simulink model "chap04_CA2"  (R2021a)
settings: Solver=FixedStepDiscrete  StartTime=0.0  StopTime=30  FixedStep=0.001  RelTol=1e-3
undefined symbols (not defined in the file): DiscIntNeverNeededParam
libraries: simulink x4
(part 2 of 3)

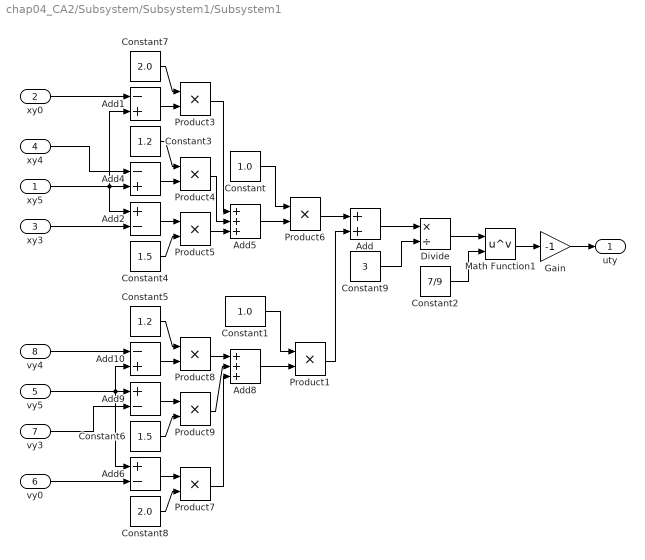
== system chap04_CA2/Subsystem/Subsystem1/Subsystem1 ==
  xy5 : Inport
  xy0 : Inport  Port=2
  xy3 : Inport  Port=3
  xy4 : Inport  Port=4
  vy5 : Inport  Port=5
  vy0 : Inport  Port=6
  vy3 : Inport  Port=7
  vy4 : Inport  Port=8
  Add : Sum
  Add1 : Sum  Inputs=-+
  Add10 : Sum  Inputs=-+
  Add2 : Sum  Inputs=+-
  Add4 : Sum  Inputs=-+
  Add5 : Sum  Inputs=+++
  Add6 : Sum  Inputs=+-
  Add8 : Sum  Inputs=+++
  Add9 : Sum  Inputs=+-
  Constant : Constant  Value=1.0
  Constant1 : Constant  Value=1.0
  Constant2 : Constant  Value=7/9
  Constant3 : Constant  Value=1.2
  Constant4 : Constant  Value=1.5
  Constant5 : Constant  Value=1.2
  Constant6 : Constant  Value=1.5
  Constant7 : Constant  Value=2.0
  Constant8 : Constant  Value=2.0
  Constant9 : Constant  Value=3
  Divide : Product  Inputs=*/
  Gain : Gain  Gain=-1
  Math Function1 : Math  Operator=pow  SignedPower=on  SaturateOnIntegerOverflow=on
  Product{1,3..9} (8 alike) : Product
  uty : Outport
  wires:
  vy0/1 -> Add6/2
  Constant8/1 -> Product7/2
  Add6/1 -> Product7/1
  Product7/1 -> Add8/3
  Product3/1 -> Add5/1
  xy0/1 -> Add1/1
  Add1/1 -> Product3/2
  Constant7/1 -> Product3/1
  Product9/1 -> Add8/2
  Product8/1 -> Add8/1
  Add9/1 -> Product9/1
  Constant6/1 -> Product9/2
  Add10/1 -> Product8/2
  Constant5/1 -> Product8/1
  Add8/1 -> Product1/2
  Product4/1 -> Add5/2
  Product5/1 -> Add5/3
  Constant3/1 -> Product4/1
  Add4/1 -> Product4/2
  xy5/1 -> Add2/1, Add4/2, Add1/2
  Constant4/1 -> Product5/2
  Product6/1 -> Add/1
  Constant/1 -> Product6/1
  Constant1/1 -> Product1/1
  Product1/1 -> Add/2
  Add2/1 -> Product5/1
  Add5/1 -> Product6/2
  xy4/1 -> Add4/1
  xy3/1 -> Add2/2
  vy3/1 -> Add9/2
  vy4/1 -> Add10/1
  vy5/1 -> Add9/1, Add6/1, Add10/2
  Math Function1/1 -> Gain/1
  Constant9/1 -> Divide/2
  Divide/1 -> Math Function1/1
  Add/1 -> Divide/1
  Constant2/1 -> Math Function1/2
  Gain/1 -> uty/1

== system chap04_CA2/Subsystem/Subsystem1/Subsystem10 ==
  utx : Inport
  uty : Inport  Port=2
  utz : Inport  Port=3
  Add : Sum
  Constant3 : Constant
  Constant4 : Constant  Value=0
  Data Store Memory : DataStoreMemory  DataStoreName=utkz5  ReadBeforeWriteMsg=warning  WriteAfterWriteMsg=warning  WriteAfterReadMsg=warning  ShowAdditionalParam=off
  Data Store Memory1 : DataStoreMemory  DataStoreName=utky5  ReadBeforeWriteMsg=warning  WriteAfterWriteMsg=warning  WriteAfterReadMsg=warning  ShowAdditionalParam=off
  Data Store Memory2 : DataStoreMemory  DataStoreName=utkx5  ReadBeforeWriteMsg=warning  WriteAfterWriteMsg=warning  WriteAfterReadMsg=warning  ShowAdditionalParam=off
  Data Store Memory3 : DataStoreMemory  DataStoreName=uc5  ReadBeforeWriteMsg=warning  WriteAfterWriteMsg=warning  WriteAfterReadMsg=warning  ShowAdditionalParam=off
  Data Store Read : DataStoreRead  DataStoreName=uc5  IndexOptions=Index vector (dialog)  Indices=1  OutputSizes=1
  Data Store Read1 : DataStoreRead  DataStoreName=utkz5  IndexOptions=Index vector (dialog)  Indices=1  OutputSizes=1
  Data Store Read2 : DataStoreRead  DataStoreName=utky5  IndexOptions=Index vector (dialog)  Indices=1  OutputSizes=1
  Data Store Read3 : DataStoreRead  DataStoreName=utkx5  IndexOptions=Index vector (dialog)  Indices=1  OutputSizes=1
  Data Store Write : DataStoreWrite  DataStoreName=uc5  IndexOptions=Index vector (dialog)  Indices=1  OutputSizes=1
  Data Store Write3 : DataStoreWrite  DataStoreName=utkx5  IndexOptions=Index vector (dialog)  Indices=1  OutputSizes=1
  Data Store Write4 : DataStoreWrite  DataStoreName=utky5  IndexOptions=Index vector (dialog)  Indices=1  OutputSizes=1
  Data Store Write5 : DataStoreWrite  DataStoreName=utkz5  IndexOptions=Index vector (dialog)  Indices=1  OutputSizes=1
  Demux : Demux  Outputs=3
  Display : Display
  MATLAB Function : MATLAB Function  TreatAsAtomicUnit=on
  Mux1 : Mux  Inputs=3
  Mux2 : Mux  Inputs=3
  Switch : Switch  Threshold=0.025
  Switch2 : Switch  Threshold=0.025
  ux : Outport
  uy : Outport  Port=2
  uz : Outport  Port=3
  wires:
  Mux2/1 -> [utk], MATLAB Function/2(utk)
  Mux1/1 -> [ut], MATLAB Function/1(u)
  Switch/1 -> Demux/1
  Data Store Read3/1 -> Mux2/1
  Data Store Read1/1 -> Mux2/3
  Data Store Read2/1 -> Mux2/2
  Demux/3 -> Data Store Write5/1, uz/1
  Demux/1 -> Data Store Write3/1, ux/1
  Add/1 -> Data Store Write/1, Display/1
  Data Store Read/1 -> Add/2
  Switch2/1 -> Add/1  "e1"
  Constant3/1 -> Switch2/1
  Constant4/1 -> Switch2/3
  MATLAB Function/1(nrom) -> Switch2/2, Switch/2
  utx/1 -> Mux1/1
  uty/1 -> Mux1/2
  utz/1 -> Mux1/3
  Demux/2 -> Data Store Write4/1, uy/1
  [ut] -> Switch/1
  [utk] -> Switch/3

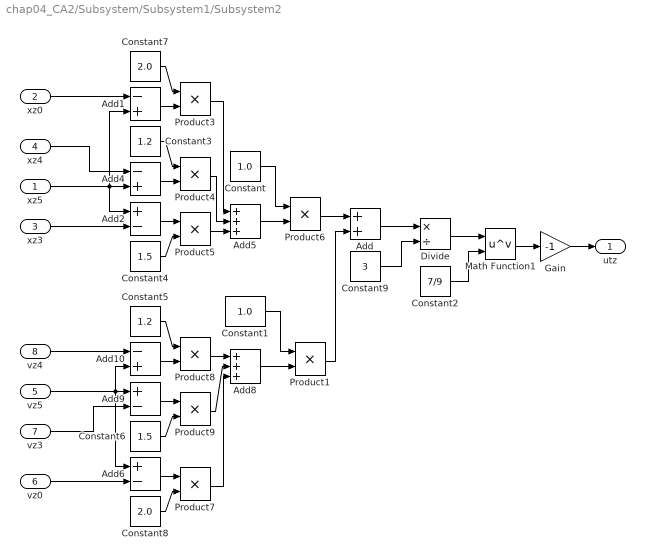
== system chap04_CA2/Subsystem/Subsystem1/Subsystem2 ==
  xz5 : Inport
  xz0 : Inport  Port=2
  xz3 : Inport  Port=3
  xz4 : Inport  Port=4
  vz5 : Inport  Port=5
  vz0 : Inport  Port=6
  vz3 : Inport  Port=7
  vz4 : Inport  Port=8
  Add : Sum
  Add1 : Sum  Inputs=-+
  Add10 : Sum  Inputs=-+
  Add2 : Sum  Inputs=+-
  Add4 : Sum  Inputs=-+
  Add5 : Sum  Inputs=+++
  Add6 : Sum  Inputs=+-
  Add8 : Sum  Inputs=+++
  Add9 : Sum  Inputs=+-
  Constant : Constant  Value=1.0
  Constant1 : Constant  Value=1.0
  Constant2 : Constant  Value=7/9
  Constant3 : Constant  Value=1.2
  Constant4 : Constant  Value=1.5
  Constant5 : Constant  Value=1.2
  Constant6 : Constant  Value=1.5
  Constant7 : Constant  Value=2.0
  Constant8 : Constant  Value=2.0
  Constant9 : Constant  Value=3
  Divide : Product  Inputs=*/
  Gain : Gain  Gain=-1
  Math Function1 : Math  Operator=pow  SignedPower=on  SaturateOnIntegerOverflow=on
  Product{1,3..9} (8 alike) : Product
  utz : Outport
  wires:
  vz5/1 -> Add10/2, Add6/1, Add9/1
  vz4/1 -> Add10/1
  vz3/1 -> Add9/2
  xz3/1 -> Add2/2
  xz4/1 -> Add4/1
  Add5/1 -> Product6/2
  Add2/1 -> Product5/1
  Product1/1 -> Add/2
  Constant1/1 -> Product1/1
  Constant/1 -> Product6/1
  Product6/1 -> Add/1
  Constant4/1 -> Product5/2
  xz5/1 -> Add1/2, Add4/2, Add2/1
  Add4/1 -> Product4/2
  Constant3/1 -> Product4/1
  Product5/1 -> Add5/3
  Product4/1 -> Add5/2
  Add8/1 -> Product1/2
  Constant5/1 -> Product8/1
  Add10/1 -> Product8/2
  Constant6/1 -> Product9/2
  Add9/1 -> Product9/1
  Product8/1 -> Add8/1
  Product9/1 -> Add8/2
  Constant7/1 -> Product3/1
  Add1/1 -> Product3/2
  xz0/1 -> Add1/1
  Product3/1 -> Add5/1
  Product7/1 -> Add8/3
  Add6/1 -> Product7/1
  Constant8/1 -> Product7/2
  vz0/1 -> Add6/2
  Math Function1/1 -> Gain/1
  Constant9/1 -> Divide/2
  Divide/1 -> Math Function1/1
  Add/1 -> Divide/1
  Constant2/1 -> Math Function1/2
  Gain/1 -> utz/1

== system chap04_CA2/Subsystem/Subsystem1/Subsystem4 ==
  vx5 : Inport
  vx0 : Inport  Port=2
  utx : Inport  Port=3
  gain : Inport  Port=4
  Add1 : Sum  Inputs=--+
  Constant : Constant  Value=0.08
  Constant2 : Constant  Value=15
  Product : Product
  Product1 : Product
  Product2 : Product
  Subsystem : Subsystem
  Subtract : Sum  Inputs=+--
  Tanh : Trigonometry  Operator=tanh
  ux : Outport
  wires:
  Add1/1 -> ux/1
  utx/1 -> [A], Subsystem/1(zt3)
  Subsystem/1(Out1) -> Subtract/3
  Product/1 -> Add1/2
  vx5/1 -> Subtract/1
  Product2/1 -> Tanh/1
  Tanh/1 -> Product/1
  gain/1 -> Product/2
  [A] -> Add1/3
  Constant2/1 -> Product2/2
  Product1/1 -> Add1/1
  Constant/1 -> Product1/1
  Subtract/1 -> Product1/2, Product2/1
  vx0/1 -> Subtract/2

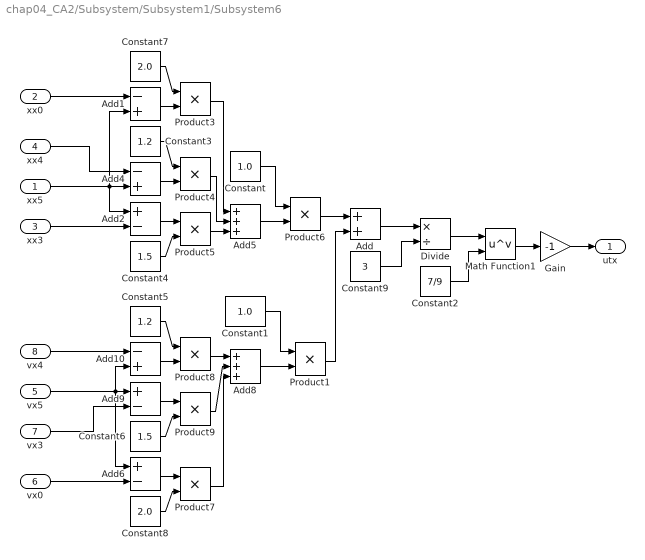
== system chap04_CA2/Subsystem/Subsystem1/Subsystem6 ==
  xx5 : Inport
  xx0 : Inport  Port=2
  xx3 : Inport  Port=3
  xx4 : Inport  Port=4
  vx5 : Inport  Port=5
  vx0 : Inport  Port=6
  vx3 : Inport  Port=7
  vx4 : Inport  Port=8
  Add : Sum
  Add1 : Sum  Inputs=-+
  Add10 : Sum  Inputs=-+
  Add2 : Sum  Inputs=+-
  Add4 : Sum  Inputs=-+
  Add5 : Sum  Inputs=+++
  Add6 : Sum  Inputs=+-
  Add8 : Sum  Inputs=+++
  Add9 : Sum  Inputs=+-
  Constant : Constant  Value=1.0
  Constant1 : Constant  Value=1.0
  Constant2 : Constant  Value=7/9
  Constant3 : Constant  Value=1.2
  Constant4 : Constant  Value=1.5
  Constant5 : Constant  Value=1.2
  Constant6 : Constant  Value=1.5
  Constant7 : Constant  Value=2.0
  Constant8 : Constant  Value=2.0
  Constant9 : Constant  Value=3
  Divide : Product  Inputs=*/
  Gain : Gain  Gain=-1
  Math Function1 : Math  Operator=pow  SignedPower=on  SaturateOnIntegerOverflow=on
  Product{1,3..9} (8 alike) : Product
  utx : Outport
  wires:
  vx5/1 -> Add10/2, Add6/1, Add9/1
  vx4/1 -> Add10/1
  vx3/1 -> Add9/2
  xx3/1 -> Add2/2
  xx4/1 -> Add4/1
  Add5/1 -> Product6/2
  Add2/1 -> Product5/1
  Product1/1 -> Add/2
  Constant1/1 -> Product1/1
  Constant/1 -> Product6/1
  Product6/1 -> Add/1
  Constant4/1 -> Product5/2
  xx5/1 -> Add1/2, Add4/2, Add2/1
  Add4/1 -> Product4/2
  Constant3/1 -> Product4/1
  Product5/1 -> Add5/3
  Product4/1 -> Add5/2
  Add8/1 -> Product1/2
  Constant5/1 -> Product8/1
  Add10/1 -> Product8/2
  Constant6/1 -> Product9/2
  Add9/1 -> Product9/1
  Product8/1 -> Add8/1
  Product9/1 -> Add8/2
  Constant7/1 -> Product3/1
  Add1/1 -> Product3/2
  xx0/1 -> Add1/1
  Product3/1 -> Add5/1
  Product7/1 -> Add8/3
  Add6/1 -> Product7/1
  Constant8/1 -> Product7/2
  vx0/1 -> Add6/2
  Math Function1/1 -> Gain/1
  Constant9/1 -> Divide/2
  Divide/1 -> Math Function1/1
  Add/1 -> Divide/1
  Constant2/1 -> Math Function1/2
  Gain/1 -> utx/1

== system chap04_CA2/Subsystem/Subsystem1/Subsystem7 ==
  vy5 : Inport
  vy0 : Inport  Port=2
  uty : Inport  Port=3
  gain : Inport  Port=4
  Add1 : Sum  Inputs=--+
  Constant : Constant  Value=0.08
  Constant2 : Constant  Value=15
  Product : Product
  Product1 : Product
  Product2 : Product
  Subsystem : Subsystem
  Subtract : Sum  Inputs=+--
  Tanh : Trigonometry  Operator=tanh
  ux : Outport
  wires:
  Subtract/1 -> Product2/1, Product1/2
  Constant/1 -> Product1/1
  Product1/1 -> Add1/1
  Constant2/1 -> Product2/2
  [A] -> Add1/3
  gain/1 -> Product/2
  Tanh/1 -> Product/1
  Product2/1 -> Tanh/1
  vy5/1 -> Subtract/1
  Product/1 -> Add1/2
  Subsystem/1(Out1) -> Subtract/3
  uty/1 -> Subsystem/1(zt3), [A]
  Add1/1 -> ux/1
  vy0/1 -> Subtract/2

== system chap04_CA2/Subsystem/Subsystem1/Subsystem8 ==
  vz5 : Inport
  vz0 : Inport  Port=2
  utz : Inport  Port=3
  gain : Inport  Port=4
  Add1 : Sum  Inputs=--+
  Constant : Constant  Value=0.08
  Constant2 : Constant  Value=15
  Product : Product
  Product1 : Product
  Product2 : Product
  Subsystem : Subsystem
  Subtract : Sum  Inputs=+--
  Tanh : Trigonometry  Operator=tanh
  ux : Outport
  wires:
  Add1/1 -> ux/1
  utz/1 -> [A], Subsystem/1(zt3)
  Subsystem/1(Out1) -> Subtract/3
  Product/1 -> Add1/2
  vz5/1 -> Subtract/1
  Product2/1 -> Tanh/1
  Tanh/1 -> Product/1
  gain/1 -> Product/2
  [A] -> Add1/3
  Constant2/1 -> Product2/2
  Product1/1 -> Add1/1
  Constant/1 -> Product1/1
  Subtract/1 -> Product1/2, Product2/1
  vz0/1 -> Subtract/2

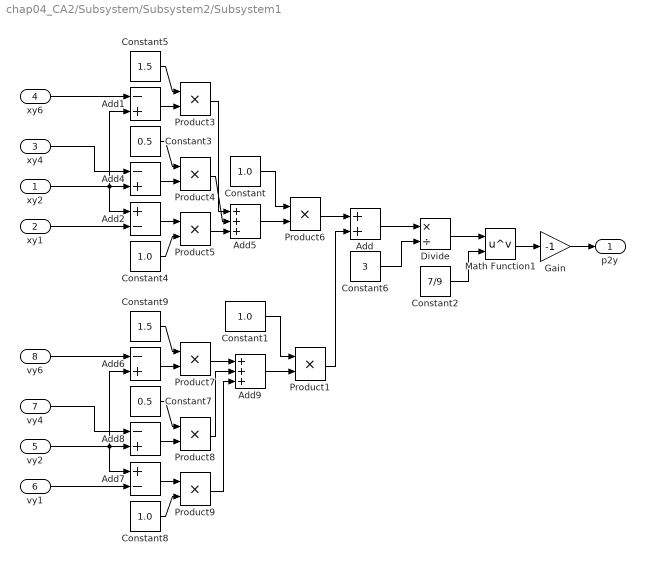
== system chap04_CA2/Subsystem/Subsystem2/Subsystem1 ==
  xy2 : Inport
  xy1 : Inport  Port=2
  xy4 : Inport  Port=3
  xy6 : Inport  Port=4
  vy2 : Inport  Port=5
  vy1 : Inport  Port=6
  vy4 : Inport  Port=7
  vy6 : Inport  Port=8
  Add : Sum
  Add{1,4,6,8} (4 alike) : Sum  Inputs=-+
  Add2 : Sum  Inputs=+-
  Add5 : Sum  Inputs=+++
  Add7 : Sum  Inputs=+-
  Add9 : Sum  Inputs=+++
  Constant{,1,4,8} (4 alike) : Constant  Value=1.0
  Constant2 : Constant  Value=7/9
  Constant3 : Constant  Value=0.5
  Constant5 : Constant  Value=1.5
  Constant6 : Constant  Value=3
  Constant7 : Constant  Value=0.5
  Constant9 : Constant  Value=1.5
  Divide : Product  Inputs=*/
  Gain : Gain  Gain=-1
  Math Function1 : Math  Operator=pow  SignedPower=on  SaturateOnIntegerOverflow=on
  Product{1,3..9} (8 alike) : Product
  p2y : Outport
  wires:
  Product8/1 -> Add9/2
  Product9/1 -> Add9/3
  Constant7/1 -> Product8/1
  Add8/1 -> Product8/2
  vy2/1 -> Add6/2, Add8/2, Add7/1
  Constant8/1 -> Product9/2
  Add7/1 -> Product9/1
  vy4/1 -> Add8/1
  vy1/1 -> Add7/2
  vy6/1 -> Add6/1
  Constant9/1 -> Product7/1
  Add6/1 -> Product7/2
  Product7/1 -> Add9/1
  Product3/1 -> Add5/1
  Add1/1 -> Product3/2
  Constant5/1 -> Product3/1
  xy6/1 -> Add1/1
  xy1/1 -> Add2/2
  xy4/1 -> Add4/1
  Add5/1 -> Product6/2
  Add2/1 -> Product5/1
  Product1/1 -> Add/2
  Constant1/1 -> Product1/1
  Constant/1 -> Product6/1
  Product6/1 -> Add/1
  Constant4/1 -> Product5/2
  xy2/1 -> Add2/1, Add4/2, Add1/2
  Add4/1 -> Product4/2
  Constant3/1 -> Product4/1
  Product5/1 -> Add5/3
  Product4/1 -> Add5/2
  Add9/1 -> Product1/2
  Math Function1/1 -> Gain/1
  Constant6/1 -> Divide/2
  Divide/1 -> Math Function1/1
  Add/1 -> Divide/1
  Constant2/1 -> Math Function1/2
  Gain/1 -> p2y/1

== system chap04_CA2/Subsystem/Subsystem2/Subsystem10 ==
  utx : Inport
  uty : Inport  Port=2
  utz : Inport  Port=3
  Add : Sum
  Constant3 : Constant
  Constant4 : Constant  Value=0
  Data Store Memory : DataStoreMemory  DataStoreName=utkz2  ReadBeforeWriteMsg=warning  WriteAfterWriteMsg=warning  WriteAfterReadMsg=warning  ShowAdditionalParam=off
  Data Store Memory1 : DataStoreMemory  DataStoreName=utky2  ReadBeforeWriteMsg=warning  WriteAfterWriteMsg=warning  WriteAfterReadMsg=warning  ShowAdditionalParam=off
  Data Store Memory2 : DataStoreMemory  DataStoreName=utkx2  ReadBeforeWriteMsg=warning  WriteAfterWriteMsg=warning  WriteAfterReadMsg=warning  ShowAdditionalParam=off
  Data Store Memory3 : DataStoreMemory  DataStoreName=uc2  ReadBeforeWriteMsg=warning  WriteAfterWriteMsg=warning  WriteAfterReadMsg=warning  ShowAdditionalParam=off
  Data Store Read : DataStoreRead  DataStoreName=uc2  IndexOptions=Index vector (dialog)  Indices=1  OutputSizes=1
  Data Store Read1 : DataStoreRead  DataStoreName=utkx2  IndexOptions=Index vector (dialog)  Indices=1  OutputSizes=1
  Data Store Read2 : DataStoreRead  DataStoreName=utky2  IndexOptions=Index vector (dialog)  Indices=1  OutputSizes=1
  Data Store Read3 : DataStoreRead  DataStoreName=utkz2  IndexOptions=Index vector (dialog)  Indices=1  OutputSizes=1
  Data Store Write : DataStoreWrite  DataStoreName=uc2  IndexOptions=Index vector (dialog)  Indices=1  OutputSizes=1
  Data Store Write1 : DataStoreWrite  DataStoreName=utkx2  IndexOptions=Index vector (dialog)  Indices=1  OutputSizes=1
  Data Store Write2 : DataStoreWrite  DataStoreName=utky2  IndexOptions=Index vector (dialog)  Indices=1  OutputSizes=1
  Data Store Write3 : DataStoreWrite  DataStoreName=utkz2  IndexOptions=Index vector (dialog)  Indices=1  OutputSizes=1
  Demux : Demux  Outputs=3
  Display : Display
  MATLAB Function : MATLAB Function  TreatAsAtomicUnit=on
  Mux1 : Mux  Inputs=3
  Mux2 : Mux  Inputs=3
  Switch : Switch  Threshold=0.025
  Switch2 : Switch  Threshold=0.025
  ux : Outport
  uy : Outport  Port=2
  uz : Outport  Port=3
  wires:
  Mux2/1 -> [utk], MATLAB Function/2(utk)
  Mux1/1 -> [ut], MATLAB Function/1(u)
  Switch/1 -> Demux/1
  Data Store Read1/1 -> Mux2/1
  Data Store Read3/1 -> Mux2/3
  Data Store Read2/1 -> Mux2/2
  Demux/3 -> Data Store Write3/1, uz/1
  Demux/1 -> Data Store Write1/1, ux/1
  Add/1 -> Data Store Write/1, Display/1
  Data Store Read/1 -> Add/2
  Switch2/1 -> Add/1  "e1"
  Constant3/1 -> Switch2/1
  Constant4/1 -> Switch2/3
  MATLAB Function/1(nrom) -> Switch2/2, Switch/2
  utx/1 -> Mux1/1
  uty/1 -> Mux1/2
  utz/1 -> Mux1/3
  Demux/2 -> Data Store Write2/1, uy/1
  [ut] -> Switch/1
  [utk] -> Switch/3

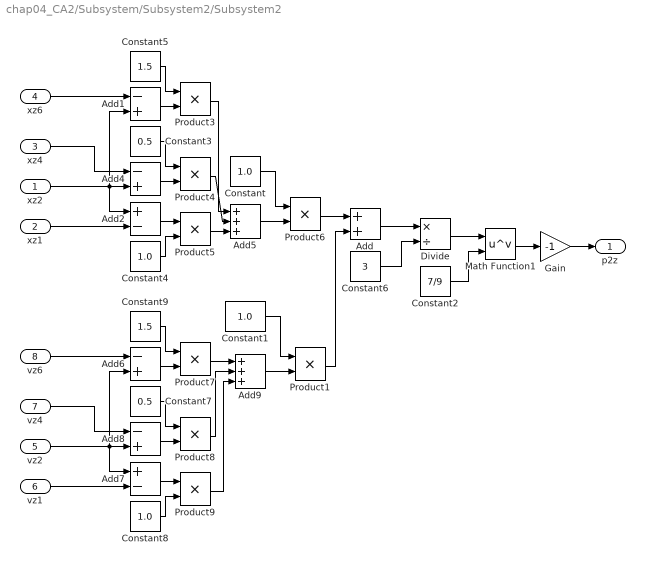
== system chap04_CA2/Subsystem/Subsystem2/Subsystem2 ==
  xz2 : Inport
  xz1 : Inport  Port=2
  xz4 : Inport  Port=3
  xz6 : Inport  Port=4
  vz2 : Inport  Port=5
  vz1 : Inport  Port=6
  vz4 : Inport  Port=7
  vz6 : Inport  Port=8
  Add : Sum
  Add{1,4,6,8} (4 alike) : Sum  Inputs=-+
  Add2 : Sum  Inputs=+-
  Add5 : Sum  Inputs=+++
  Add7 : Sum  Inputs=+-
  Add9 : Sum  Inputs=+++
  Constant{,1,4,8} (4 alike) : Constant  Value=1.0
  Constant2 : Constant  Value=7/9
  Constant3 : Constant  Value=0.5
  Constant5 : Constant  Value=1.5
  Constant6 : Constant  Value=3
  Constant7 : Constant  Value=0.5
  Constant9 : Constant  Value=1.5
  Divide : Product  Inputs=*/
  Gain : Gain  Gain=-1
  Math Function1 : Math  Operator=pow  SignedPower=on  SaturateOnIntegerOverflow=on
  Product{1,3..9} (8 alike) : Product
  p2z : Outport
  wires:
  Add9/1 -> Product1/2
  Product4/1 -> Add5/2
  Product5/1 -> Add5/3
  Constant3/1 -> Product4/1
  Add4/1 -> Product4/2
  xz2/1 -> Add1/2, Add4/2, Add2/1
  Constant4/1 -> Product5/2
  Product6/1 -> Add/1
  Constant/1 -> Product6/1
  Constant1/1 -> Product1/1
  Product1/1 -> Add/2
  Add2/1 -> Product5/1
  Add5/1 -> Product6/2
  xz4/1 -> Add4/1
  xz1/1 -> Add2/2
  xz6/1 -> Add1/1
  Constant5/1 -> Product3/1
  Add1/1 -> Product3/2
  Product3/1 -> Add5/1
  Product7/1 -> Add9/1
  Add6/1 -> Product7/2
  Constant9/1 -> Product7/1
  vz6/1 -> Add6/1
  vz1/1 -> Add7/2
  vz4/1 -> Add8/1
  Add7/1 -> Product9/1
  Constant8/1 -> Product9/2
  vz2/1 -> Add7/1, Add8/2, Add6/2
  Add8/1 -> Product8/2
  Constant7/1 -> Product8/1
  Product9/1 -> Add9/3
  Product8/1 -> Add9/2
  Math Function1/1 -> Gain/1
  Constant6/1 -> Divide/2
  Divide/1 -> Math Function1/1
  Add/1 -> Divide/1
  Constant2/1 -> Math Function1/2
  Gain/1 -> p2z/1

== system chap04_CA2/Subsystem/Subsystem2/Subsystem4 ==
  vx1 : Inport
  utx : Inport  Port=2
  gain : Inport  Port=3
  Add1 : Sum  Inputs=--+
  Constant : Constant  Value=0.08
  Constant2 : Constant  Value=15
  Product : Product
  Product1 : Product
  Product2 : Product
  Subsystem : Subsystem
  Subtract : Sum  Inputs=+-
  Tanh : Trigonometry  Operator=tanh
  ux : Outport
  wires:
  Add1/1 -> ux/1
  utx/1 -> [A], Subsystem/1(zt3)
  Subsystem/1(Out1) -> Subtract/2
  Product/1 -> Add1/2
  vx1/1 -> Subtract/1
  Product2/1 -> Tanh/1
  Tanh/1 -> Product/1
  gain/1 -> Product/2
  [A] -> Add1/3
  Constant2/1 -> Product2/2
  Product1/1 -> Add1/1
  Constant/1 -> Product1/1
  Subtract/1 -> Product1/2, Product2/1

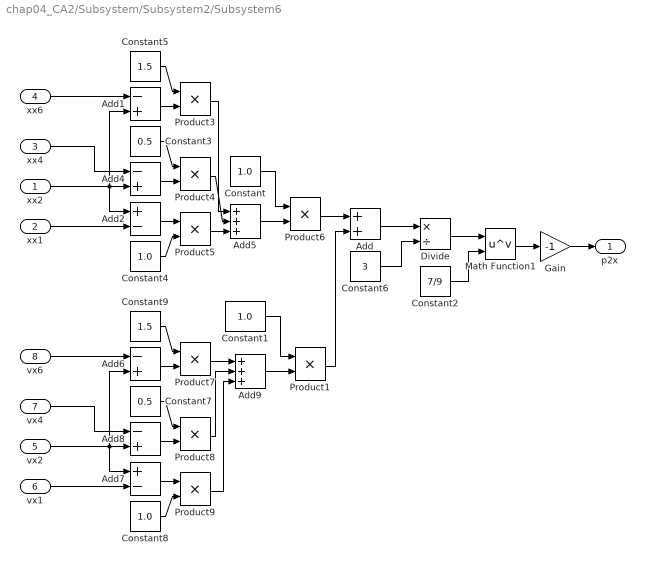
== system chap04_CA2/Subsystem/Subsystem2/Subsystem6 ==
  xx2 : Inport
  xx1 : Inport  Port=2
  xx4 : Inport  Port=3
  xx6 : Inport  Port=4
  vx2 : Inport  Port=5
  vx1 : Inport  Port=6
  vx4 : Inport  Port=7
  vx6 : Inport  Port=8
  Add : Sum
  Add{1,4,6,8} (4 alike) : Sum  Inputs=-+
  Add2 : Sum  Inputs=+-
  Add5 : Sum  Inputs=+++
  Add7 : Sum  Inputs=+-
  Add9 : Sum  Inputs=+++
  Constant{,1,4,8} (4 alike) : Constant  Value=1.0
  Constant2 : Constant  Value=7/9
  Constant3 : Constant  Value=0.5
  Constant5 : Constant  Value=1.5
  Constant6 : Constant  Value=3
  Constant7 : Constant  Value=0.5
  Constant9 : Constant  Value=1.5
  Divide : Product  Inputs=*/
  Gain : Gain  Gain=-1
  Math Function1 : Math  Operator=pow  SignedPower=on  SaturateOnIntegerOverflow=on
  Product{1,3..9} (8 alike) : Product
  p2x : Outport
  wires:
  Add9/1 -> Product1/2
  Product4/1 -> Add5/2
  Product5/1 -> Add5/3
  Constant3/1 -> Product4/1
  Add4/1 -> Product4/2
  xx2/1 -> Add1/2, Add4/2, Add2/1
  Constant4/1 -> Product5/2
  Product6/1 -> Add/1
  Constant/1 -> Product6/1
  Constant1/1 -> Product1/1
  Product1/1 -> Add/2
  Add2/1 -> Product5/1
  Add5/1 -> Product6/2
  xx4/1 -> Add4/1
  xx1/1 -> Add2/2
  xx6/1 -> Add1/1
  Constant5/1 -> Product3/1
  Add1/1 -> Product3/2
  Product3/1 -> Add5/1
  Product7/1 -> Add9/1
  Add6/1 -> Product7/2
  Constant9/1 -> Product7/1
  vx6/1 -> Add6/1
  vx1/1 -> Add7/2
  vx4/1 -> Add8/1
  Add7/1 -> Product9/1
  Constant8/1 -> Product9/2
  vx2/1 -> Add7/1, Add8/2, Add6/2
  Add8/1 -> Product8/2
  Constant7/1 -> Product8/1
  Product9/1 -> Add9/3
  Product8/1 -> Add9/2
  Math Function1/1 -> Gain/1
  Constant6/1 -> Divide/2
  Divide/1 -> Math Function1/1
  Add/1 -> Divide/1
  Constant2/1 -> Math Function1/2
  Gain/1 -> p2x/1

== system chap04_CA2/Subsystem/Subsystem2/Subsystem7 ==
  vy1 : Inport
  uty : Inport  Port=2
  gain : Inport  Port=3
  Add1 : Sum  Inputs=--+
  Constant : Constant  Value=0.08
  Constant2 : Constant  Value=15
  Product : Product
  Product1 : Product
  Product2 : Product
  Subsystem : Subsystem
  Subtract : Sum  Inputs=+-
  Tanh : Trigonometry  Operator=tanh
  ux : Outport
  wires:
  Subtract/1 -> Product2/1, Product1/2
  Constant/1 -> Product1/1
  Product1/1 -> Add1/1
  Constant2/1 -> Product2/2
  [A] -> Add1/3
  gain/1 -> Product/2
  Tanh/1 -> Product/1
  Product2/1 -> Tanh/1
  vy1/1 -> Subtract/1
  Product/1 -> Add1/2
  Subsystem/1(Out1) -> Subtract/2
  uty/1 -> Subsystem/1(zt3), [A]
  Add1/1 -> ux/1

== system chap04_CA2/Subsystem/Subsystem2/Subsystem8 ==
  vz1 : Inport
  utz : Inport  Port=2
  gain : Inport  Port=3
  Add1 : Sum  Inputs=--+
  Constant : Constant  Value=0.08
  Constant2 : Constant  Value=15
  Product : Product
  Product1 : Product
  Product2 : Product
  Subsystem : Subsystem
  Subtract : Sum  Inputs=+-
  Tanh : Trigonometry  Operator=tanh
  ux : Outport
  wires:
  Add1/1 -> ux/1
  utz/1 -> [A], Subsystem/1(zt3)
  Subsystem/1(Out1) -> Subtract/2
  Product/1 -> Add1/2
  vz1/1 -> Subtract/1
  Product2/1 -> Tanh/1
  Tanh/1 -> Product/1
  gain/1 -> Product/2
  [A] -> Add1/3
  Constant2/1 -> Product2/2
  Product1/1 -> Add1/1
  Constant/1 -> Product1/1
  Subtract/1 -> Product1/2, Product2/1

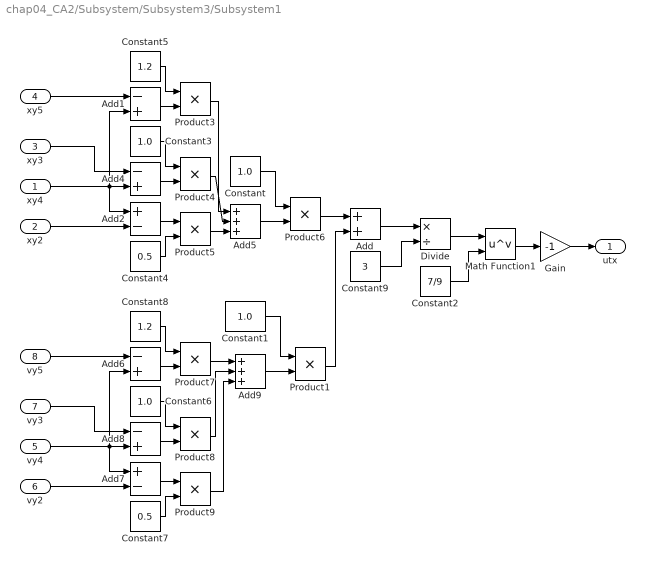
== system chap04_CA2/Subsystem/Subsystem3/Subsystem1 ==
  xy4 : Inport
  xy2 : Inport  Port=2
  xy3 : Inport  Port=3
  xy5 : Inport  Port=4
  vy4 : Inport  Port=5
  vy2 : Inport  Port=6
  vy3 : Inport  Port=7
  vy5 : Inport  Port=8
  Add : Sum
  Add{1,4,6,8} (4 alike) : Sum  Inputs=-+
  Add2 : Sum  Inputs=+-
  Add5 : Sum  Inputs=+++
  Add7 : Sum  Inputs=+-
  Add9 : Sum  Inputs=+++
  Constant{,1,3,6} (4 alike) : Constant  Value=1.0
  Constant2 : Constant  Value=7/9
  Constant4 : Constant  Value=0.5
  Constant5 : Constant  Value=1.2
  Constant7 : Constant  Value=0.5
  Constant8 : Constant  Value=1.2
  Constant9 : Constant  Value=3
  Divide : Product  Inputs=*/
  Gain : Gain  Gain=-1
  Math Function1 : Math  Operator=pow  SignedPower=on  SaturateOnIntegerOverflow=on
  Product{1,3..9} (8 alike) : Product
  utx : Outport
  wires:
  Add9/1 -> Product1/2
  Product4/1 -> Add5/2
  Product5/1 -> Add5/3
  Constant3/1 -> Product4/1
  Add4/1 -> Product4/2
  xy4/1 -> Add1/2, Add4/2, Add2/1
  Constant4/1 -> Product5/2
  Product6/1 -> Add/1
  Constant/1 -> Product6/1
  Constant1/1 -> Product1/1
  Product1/1 -> Add/2
  Add2/1 -> Product5/1
  Add5/1 -> Product6/2
  xy3/1 -> Add4/1
  xy2/1 -> Add2/2
  xy5/1 -> Add1/1
  Constant5/1 -> Product3/1
  Add1/1 -> Product3/2
  Product3/1 -> Add5/1
  Product7/1 -> Add9/1
  Add6/1 -> Product7/2
  Constant8/1 -> Product7/1
  vy5/1 -> Add6/1
  vy2/1 -> Add7/2
  vy3/1 -> Add8/1
  Add7/1 -> Product9/1
  Constant7/1 -> Product9/2
  vy4/1 -> Add7/1, Add8/2, Add6/2
  Add8/1 -> Product8/2
  Constant6/1 -> Product8/1
  Product9/1 -> Add9/3
  Product8/1 -> Add9/2
  Math Function1/1 -> Gain/1
  Constant9/1 -> Divide/2
  Divide/1 -> Math Function1/1
  Add/1 -> Divide/1
  Constant2/1 -> Math Function1/2
  Gain/1 -> utx/1

== system chap04_CA2/Subsystem/Subsystem3/Subsystem10 ==
  utx : Inport
  uty : Inport  Port=2
  utz : Inport  Port=3
  Add : Sum
  Constant3 : Constant
  Constant4 : Constant  Value=0
  Data Store Memory : DataStoreMemory  DataStoreName=utkz4  ReadBeforeWriteMsg=warning  WriteAfterWriteMsg=warning  WriteAfterReadMsg=warning  ShowAdditionalParam=off
  Data Store Memory1 : DataStoreMemory  DataStoreName=utky4  ReadBeforeWriteMsg=warning  WriteAfterWriteMsg=warning  WriteAfterReadMsg=warning  ShowAdditionalParam=off
  Data Store Memory2 : DataStoreMemory  DataStoreName=utkx4  ReadBeforeWriteMsg=warning  WriteAfterWriteMsg=warning  WriteAfterReadMsg=warning  ShowAdditionalParam=off
  Data Store Memory3 : DataStoreMemory  DataStoreName=uc4  ReadBeforeWriteMsg=warning  WriteAfterWriteMsg=warning  WriteAfterReadMsg=warning  ShowAdditionalParam=off
  Data Store Read : DataStoreRead  DataStoreName=uc4  IndexOptions=Index vector (dialog)  Indices=1  OutputSizes=1
  Data Store Read1 : DataStoreRead  DataStoreName=utkz4  IndexOptions=Index vector (dialog)  Indices=1  OutputSizes=1
  Data Store Read2 : DataStoreRead  DataStoreName=utky4  IndexOptions=Index vector (dialog)  Indices=1  OutputSizes=1
  Data Store Read3 : DataStoreRead  DataStoreName=utkx4  IndexOptions=Index vector (dialog)  Indices=1  OutputSizes=1
  Data Store Write : DataStoreWrite  DataStoreName=uc4  IndexOptions=Index vector (dialog)  Indices=1  OutputSizes=1
  Data Store Write3 : DataStoreWrite  DataStoreName=utkx4  IndexOptions=Index vector (dialog)  Indices=1  OutputSizes=1
  Data Store Write4 : DataStoreWrite  DataStoreName=utky4  IndexOptions=Index vector (dialog)  Indices=1  OutputSizes=1
  Data Store Write5 : DataStoreWrite  DataStoreName=utkz4  IndexOptions=Index vector (dialog)  Indices=1  OutputSizes=1
  Demux : Demux  Outputs=3
  Display : Display
  MATLAB Function : MATLAB Function  TreatAsAtomicUnit=on
  Mux1 : Mux  Inputs=3
  Mux2 : Mux  Inputs=3
  Switch : Switch  Threshold=0.025
  Switch2 : Switch  Threshold=0.025
  ux : Outport
  uy : Outport  Port=2
  uz : Outport  Port=3
  wires:
  Mux2/1 -> [utk], MATLAB Function/2(utk)
  Mux1/1 -> [ut], MATLAB Function/1(u)
  Switch/1 -> Demux/1
  Data Store Read3/1 -> Mux2/1
  Data Store Read1/1 -> Mux2/3
  Data Store Read2/1 -> Mux2/2
  Demux/3 -> Data Store Write5/1, uz/1
  Demux/1 -> Data Store Write3/1, ux/1
  Add/1 -> Data Store Write/1, Display/1
  Data Store Read/1 -> Add/2
  Switch2/1 -> Add/1  "e1"
  Constant3/1 -> Switch2/1
  Constant4/1 -> Switch2/3
  MATLAB Function/1(nrom) -> Switch2/2, Switch/2
  utx/1 -> Mux1/1
  uty/1 -> Mux1/2
  utz/1 -> Mux1/3
  Demux/2 -> Data Store Write4/1, uy/1
  [ut] -> Switch/1
  [utk] -> Switch/3

== system chap04_CA2/Subsystem/Subsystem3/Subsystem2 ==
  xz4 : Inport
  xx2 : Inport  Port=2
  xz3 : Inport  Port=3
  xz5 : Inport  Port=4
  vz4 : Inport  Port=5
  vz2 : Inport  Port=6
  vz3 : Inport  Port=7
  vz5 : Inport  Port=8
  Add : Sum
  Add{1,4,6,8} (4 alike) : Sum  Inputs=-+
  Add2 : Sum  Inputs=+-
  Add5 : Sum  Inputs=+++
  Add7 : Sum  Inputs=+-
  Add9 : Sum  Inputs=+++
  Constant{,1,3,6} (4 alike) : Constant  Value=1.0
  Constant2 : Constant  Value=7/9
  Constant4 : Constant  Value=0.5
  Constant5 : Constant  Value=1.2
  Constant7 : Constant  Value=0.5
  Constant8 : Constant  Value=1.2
  Constant9 : Constant  Value=3
  Divide : Product  Inputs=*/
  Gain : Gain  Gain=-1
  Math Function1 : Math  Operator=pow  SignedPower=on  SaturateOnIntegerOverflow=on
  Product{1,3..9} (8 alike) : Product
  utx : Outport
  wires:
  Product8/1 -> Add9/2
  Product9/1 -> Add9/3
  Constant6/1 -> Product8/1
  Add8/1 -> Product8/2
  vz4/1 -> Add6/2, Add8/2, Add7/1
  Constant7/1 -> Product9/2
  Add7/1 -> Product9/1
  vz3/1 -> Add8/1
  vz2/1 -> Add7/2
  vz5/1 -> Add6/1
  Constant8/1 -> Product7/1
  Add6/1 -> Product7/2
  Product7/1 -> Add9/1
  Product3/1 -> Add5/1
  Add1/1 -> Product3/2
  Constant5/1 -> Product3/1
  xz5/1 -> Add1/1
  xx2/1 -> Add2/2
  xz3/1 -> Add4/1
  Add5/1 -> Product6/2
  Add2/1 -> Product5/1
  Product1/1 -> Add/2
  Constant1/1 -> Product1/1
  Constant/1 -> Product6/1
  Product6/1 -> Add/1
  Constant4/1 -> Product5/2
  xz4/1 -> Add2/1, Add4/2, Add1/2
  Add4/1 -> Product4/2
  Constant3/1 -> Product4/1
  Product5/1 -> Add5/3
  Product4/1 -> Add5/2
  Add9/1 -> Product1/2
  Math Function1/1 -> Gain/1
  Constant9/1 -> Divide/2
  Divide/1 -> Math Function1/1
  Add/1 -> Divide/1
  Constant2/1 -> Math Function1/2
  Gain/1 -> utx/1

== system chap04_CA2/Subsystem/Subsystem3/Subsystem4 ==
  vx4 : Inport
  utx : Inport  Port=2
  gain : Inport  Port=3
  Add1 : Sum  Inputs=--+
  Constant : Constant  Value=0.08
  Constant2 : Constant  Value=15
  Product : Product
  Product1 : Product
  Product2 : Product
  Subsystem : Subsystem
  Subtract : Sum  Inputs=+-
  Tanh : Trigonometry  Operator=tanh
  ux : Outport
  wires:
  Add1/1 -> ux/1
  utx/1 -> [A], Subsystem/1(zt3)
  Subsystem/1(Out1) -> Subtract/2
  Product/1 -> Add1/2
  vx4/1 -> Subtract/1
  Product2/1 -> Tanh/1
  Tanh/1 -> Product/1
  gain/1 -> Product/2
  [A] -> Add1/3
  Constant2/1 -> Product2/2
  Product1/1 -> Add1/1
  Constant/1 -> Product1/1
  Subtract/1 -> Product1/2, Product2/1

== system chap04_CA2/Subsystem/Subsystem3/Subsystem6 ==
  xx4 : Inport
  xx2 : Inport  Port=2
  xx3 : Inport  Port=3
  xx5 : Inport  Port=4
  vx4 : Inport  Port=5
  vx2 : Inport  Port=6
  vx3 : Inport  Port=7
  vx5 : Inport  Port=8
  Add : Sum
  Add{1,4,6,8} (4 alike) : Sum  Inputs=-+
  Add2 : Sum  Inputs=+-
  Add5 : Sum  Inputs=+++
  Add7 : Sum  Inputs=+-
  Add9 : Sum  Inputs=+++
  Constant{,1,3,6} (4 alike) : Constant  Value=1.0
  Constant2 : Constant  Value=7/9
  Constant4 : Constant  Value=0.5
  Constant5 : Constant  Value=1.2
  Constant7 : Constant  Value=0.5
  Constant8 : Constant  Value=1.2
  Constant9 : Constant  Value=3
  Divide : Product  Inputs=*/
  Gain : Gain  Gain=-1
  Math Function1 : Math  Operator=pow  SignedPower=on  SaturateOnIntegerOverflow=on
  Product{1,3..9} (8 alike) : Product
  utx : Outport
  wires:
  Product8/1 -> Add9/2
  Product9/1 -> Add9/3
  Constant6/1 -> Product8/1
  Add8/1 -> Product8/2
  vx4/1 -> Add6/2, Add8/2, Add7/1
  Constant7/1 -> Product9/2
  Add7/1 -> Product9/1
  vx3/1 -> Add8/1
  vx2/1 -> Add7/2
  vx5/1 -> Add6/1
  Constant8/1 -> Product7/1
  Add6/1 -> Product7/2
  Product7/1 -> Add9/1
  Product3/1 -> Add5/1
  Add1/1 -> Product3/2
  Constant5/1 -> Product3/1
  xx5/1 -> Add1/1
  xx2/1 -> Add2/2
  xx3/1 -> Add4/1
  Add5/1 -> Product6/2
  Add2/1 -> Product5/1
  Product1/1 -> Add/2
  Constant1/1 -> Product1/1
  Constant/1 -> Product6/1
  Product6/1 -> Add/1
  Constant4/1 -> Product5/2
  xx4/1 -> Add2/1, Add4/2, Add1/2
  Add4/1 -> Product4/2
  Constant3/1 -> Product4/1
  Product5/1 -> Add5/3
  Product4/1 -> Add5/2
  Add9/1 -> Product1/2
  Math Function1/1 -> Gain/1
  Constant9/1 -> Divide/2
  Divide/1 -> Math Function1/1
  Add/1 -> Divide/1
  Constant2/1 -> Math Function1/2
  Gain/1 -> utx/1

== system chap04_CA2/Subsystem/Subsystem3/Subsystem7 ==
  vy4 : Inport
  uty : Inport  Port=2
  gain : Inport  Port=3
  Add1 : Sum  Inputs=--+
  Constant : Constant  Value=0.08
  Constant2 : Constant  Value=15
  Product : Product
  Product1 : Product
  Product2 : Product
  Subsystem : Subsystem
  Subtract : Sum  Inputs=+-
  Tanh : Trigonometry  Operator=tanh
  ux : Outport
  wires:
  Subtract/1 -> Product2/1, Product1/2
  Constant/1 -> Product1/1
  Product1/1 -> Add1/1
  Constant2/1 -> Product2/2
  [A] -> Add1/3
  gain/1 -> Product/2
  Tanh/1 -> Product/1
  Product2/1 -> Tanh/1
  vy4/1 -> Subtract/1
  Product/1 -> Add1/2
  Subsystem/1(Out1) -> Subtract/2
  uty/1 -> Subsystem/1(zt3), [A]
  Add1/1 -> ux/1

== system chap04_CA2/Subsystem/Subsystem3/Subsystem8 ==
  vz4 : Inport
  utz : Inport  Port=2
  gain : Inport  Port=3
  Add1 : Sum  Inputs=--+
  Constant : Constant  Value=0.08
  Constant2 : Constant  Value=15
  Product : Product
  Product1 : Product
  Product2 : Product
  Subsystem : Subsystem
  Subtract : Sum  Inputs=+-
  Tanh : Trigonometry  Operator=tanh
  ux : Outport
  wires:
  Add1/1 -> ux/1
  utz/1 -> [A], Subsystem/1(zt3)
  Subsystem/1(Out1) -> Subtract/2
  Product/1 -> Add1/2
  vz4/1 -> Subtract/1
  Product2/1 -> Tanh/1
  Tanh/1 -> Product/1
  gain/1 -> Product/2
  [A] -> Add1/3
  Constant2/1 -> Product2/2
  Product1/1 -> Add1/1
  Constant/1 -> Product1/1
  Subtract/1 -> Product1/2, Product2/1

== system chap04_CA2/Subsystem/Subsystem4/Subsystem1 ==
  xx6 : Inport
  xx0 : Inport  Port=2
  xx1 : Inport  Port=3
  xx2 : Inport  Port=4
  vx6 : Inport  Port=5
  vx0 : Inport  Port=6
  vx1 : Inport  Port=7
  vx2 : Inport  Port=8
  Add : Sum
  Add1 : Sum  Inputs=-+
  Add10 : Sum  Inputs=-+
  Add2 : Sum  Inputs=+-
  Add4 : Sum  Inputs=-+
  Add5 : Sum  Inputs=+++
  Add6 : Sum  Inputs=+-
  Add8 : Sum  Inputs=+++
  Add9 : Sum  Inputs=+-
  Constant : Constant  Value=1.0
  Constant1 : Constant  Value=1.0
  Constant2 : Constant  Value=7/9
  Constant3 : Constant  Value=1.2
  Constant4 : Constant  Value=1.5
  Constant5 : Constant  Value=1.5
  Constant6 : Constant  Value=1.2
  Constant7 : Constant  Value=2.0
  Constant8 : Constant  Value=2.0
  Constant9 : Constant  Value=3
  Divide : Product  Inputs=*/
  Gain : Gain  Gain=-1
  Math Function1 : Math  Operator=pow  SignedPower=on  SaturateOnIntegerOverflow=on
  Product{1,3..9} (8 alike) : Product
  utx : Outport
  wires:
  Product7/1 -> Add8/3
  Add6/1 -> Product7/1
  Constant8/1 -> Product7/2
  vx0/1 -> Add6/2
  Product3/1 -> Add5/1
  Add1/1 -> Product3/2
  Constant7/1 -> Product3/1
  xx0/1 -> Add1/1
  vx6/1 -> Add10/2, Add9/1, Add6/1
  vx2/1 -> Add10/1
  vx1/1 -> Add9/2
  xx1/1 -> Add2/2
  xx2/1 -> Add4/1
  Add5/1 -> Product6/2
  Add2/1 -> Product5/1
  Product1/1 -> Add/2
  Constant1/1 -> Product1/1
  Constant/1 -> Product6/1
  Product6/1 -> Add/1
  Constant3/1 -> Product5/2
  xx6/1 -> Add4/2, Add2/1, Add1/2
  Add4/1 -> Product4/2
  Constant4/1 -> Product4/1
  Product5/1 -> Add5/3
  Product4/1 -> Add5/2
  Add8/1 -> Product1/2
  Constant5/1 -> Product8/1
  Add10/1 -> Product8/2
  Constant6/1 -> Product9/2
  Add9/1 -> Product9/1
  Product8/1 -> Add8/1
  Product9/1 -> Add8/2
  Math Function1/1 -> Gain/1
  Constant9/1 -> Divide/2
  Divide/1 -> Math Function1/1
  Add/1 -> Divide/1
  Constant2/1 -> Math Function1/2
  Gain/1 -> utx/1

== system chap04_CA2/Subsystem/Subsystem4/Subsystem10 ==
  utx : Inport
  uty : Inport  Port=2
  utz : Inport  Port=3
  Add : Sum
  Constant3 : Constant
  Constant4 : Constant  Value=0
  Data Store Memory : DataStoreMemory  DataStoreName=utkz6  ReadBeforeWriteMsg=warning  WriteAfterWriteMsg=warning  WriteAfterReadMsg=warning  ShowAdditionalParam=off
  Data Store Memory1 : DataStoreMemory  DataStoreName=utky6  ReadBeforeWriteMsg=warning  WriteAfterWriteMsg=warning  WriteAfterReadMsg=warning  ShowAdditionalParam=off
  Data Store Memory2 : DataStoreMemory  DataStoreName=utkx6  ReadBeforeWriteMsg=warning  WriteAfterWriteMsg=warning  WriteAfterReadMsg=warning  ShowAdditionalParam=off
  Data Store Memory3 : DataStoreMemory  DataStoreName=uc6  ReadBeforeWriteMsg=warning  WriteAfterWriteMsg=warning  WriteAfterReadMsg=warning  ShowAdditionalParam=off
  Data Store Read : DataStoreRead  DataStoreName=uc6  IndexOptions=Index vector (dialog)  Indices=1  OutputSizes=1
  Data Store Read4 : DataStoreRead  DataStoreName=utkx6  IndexOptions=Index vector (dialog)  Indices=1  OutputSizes=1
  Data Store Read5 : DataStoreRead  DataStoreName=utky6  IndexOptions=Index vector (dialog)  Indices=1  OutputSizes=1
  Data Store Read6 : DataStoreRead  DataStoreName=utkz6  IndexOptions=Index vector (dialog)  Indices=1  OutputSizes=1
  Data Store Write : DataStoreWrite  DataStoreName=uc6  IndexOptions=Index vector (dialog)  Indices=1  OutputSizes=1
  Data Store Write1 : DataStoreWrite  DataStoreName=utkx6  IndexOptions=Index vector (dialog)  Indices=1  OutputSizes=1
  Data Store Write2 : DataStoreWrite  DataStoreName=utky6  IndexOptions=Index vector (dialog)  Indices=1  OutputSizes=1
  Data Store Write3 : DataStoreWrite  DataStoreName=utkz6  IndexOptions=Index vector (dialog)  Indices=1  OutputSizes=1
  Demux : Demux  Outputs=3
  Display : Display
  MATLAB Function : MATLAB Function  TreatAsAtomicUnit=on
  Mux1 : Mux  Inputs=3
  Mux2 : Mux  Inputs=3
  Switch : Switch  Threshold=0.025
  Switch2 : Switch  Threshold=0.025
  ux : Outport
  uy : Outport  Port=2
  uz : Outport  Port=3
  wires:
  Mux2/1 -> [utk], MATLAB Function/2(utk)
  Mux1/1 -> [ut], MATLAB Function/1(u)
  Switch/1 -> Demux/1
  Data Store Read4/1 -> Mux2/1
  Data Store Read6/1 -> Mux2/3
  Data Store Read5/1 -> Mux2/2
  Demux/3 -> Data Store Write3/1, uz/1
  Demux/1 -> Data Store Write1/1, ux/1
  Add/1 -> Data Store Write/1, Display/1
  Data Store Read/1 -> Add/2
  Switch2/1 -> Add/1  "e1"
  Constant3/1 -> Switch2/1
  Constant4/1 -> Switch2/3
  MATLAB Function/1(nrom) -> Switch2/2, Switch/2
  utx/1 -> Mux1/1
  uty/1 -> Mux1/2
  utz/1 -> Mux1/3
  Demux/2 -> Data Store Write2/1, uy/1
  [ut] -> Switch/1
  [utk] -> Switch/3

== system chap04_CA2/Subsystem/Subsystem4/Subsystem2 ==
  xx6 : Inport
  xx0 : Inport  Port=2
  xx1 : Inport  Port=3
  xx2 : Inport  Port=4
  vx6 : Inport  Port=5
  vx0 : Inport  Port=6
  vx1 : Inport  Port=7
  vx2 : Inport  Port=8
  Add : Sum
  Add1 : Sum  Inputs=-+
  Add10 : Sum  Inputs=-+
  Add2 : Sum  Inputs=+-
  Add4 : Sum  Inputs=-+
  Add5 : Sum  Inputs=+++
  Add6 : Sum  Inputs=+-
  Add8 : Sum  Inputs=+++
  Add9 : Sum  Inputs=+-
  Constant : Constant  Value=1.0
  Constant1 : Constant  Value=1.0
  Constant2 : Constant  Value=7/9
  Constant3 : Constant  Value=1.2
  Constant4 : Constant  Value=1.5
  Constant5 : Constant  Value=1.5
  Constant6 : Constant  Value=1.2
  Constant7 : Constant  Value=2.0
  Constant8 : Constant  Value=2.0
  Constant9 : Constant  Value=3
  Divide : Product  Inputs=*/
  Gain : Gain  Gain=-1
  Math Function1 : Math  Operator=pow  SignedPower=on  SaturateOnIntegerOverflow=on
  Product{1,3..9} (8 alike) : Product
  utx : Outport
  wires:
  Product9/1 -> Add8/2
  Product8/1 -> Add8/1
  Add9/1 -> Product9/1
  Constant6/1 -> Product9/2
  Add10/1 -> Product8/2
  Constant5/1 -> Product8/1
  Add8/1 -> Product1/2
  Product4/1 -> Add5/2
  Product5/1 -> Add5/3
  Constant4/1 -> Product4/1
  Add4/1 -> Product4/2
  xx6/1 -> Add1/2, Add2/1, Add4/2
  Constant3/1 -> Product5/2
  Product6/1 -> Add/1
  Constant/1 -> Product6/1
  Constant1/1 -> Product1/1
  Product1/1 -> Add/2
  Add2/1 -> Product5/1
  Add5/1 -> Product6/2
  xx2/1 -> Add4/1
  xx1/1 -> Add2/2
  vx1/1 -> Add9/2
  vx2/1 -> Add10/1
  vx6/1 -> Add6/1, Add9/1, Add10/2
  xx0/1 -> Add1/1
  Constant7/1 -> Product3/1
  Add1/1 -> Product3/2
  Product3/1 -> Add5/1
  vx0/1 -> Add6/2
  Constant8/1 -> Product7/2
  Add6/1 -> Product7/1
  Product7/1 -> Add8/3
  Math Function1/1 -> Gain/1
  Constant9/1 -> Divide/2
  Divide/1 -> Math Function1/1
  Add/1 -> Divide/1
  Constant2/1 -> Math Function1/2
  Gain/1 -> utx/1

== system chap04_CA2/Subsystem/Subsystem4/Subsystem4 ==
  vx6 : Inport
  vx0 : Inport  Port=2
  utx : Inport  Port=3
  gain : Inport  Port=4
  Add1 : Sum  Inputs=--+
  Constant : Constant  Value=0.08
  Constant2 : Constant  Value=15
  Product : Product
  Product1 : Product
  Product2 : Product
  Subsystem : Subsystem
  Subtract : Sum  Inputs=+--
  Tanh : Trigonometry  Operator=tanh
  ux : Outport
  wires:
  Add1/1 -> ux/1
  utx/1 -> [A], Subsystem/1(zt3)
  Subsystem/1(Out1) -> Subtract/3
  Product/1 -> Add1/2
  vx6/1 -> Subtract/1
  Product2/1 -> Tanh/1
  Tanh/1 -> Product/1
  gain/1 -> Product/2
  [A] -> Add1/3
  Constant2/1 -> Product2/2
  Product1/1 -> Add1/1
  Constant/1 -> Product1/1
  Subtract/1 -> Product1/2, Product2/1
  vx0/1 -> Subtract/2

== system chap04_CA2/Subsystem/Subsystem4/Subsystem6 ==
  xx6 : Inport
  xx0 : Inport  Port=2
  xx1 : Inport  Port=3
  xx2 : Inport  Port=4
  vx6 : Inport  Port=5
  vx0 : Inport  Port=6
  vx1 : Inport  Port=7
  vx2 : Inport  Port=8
  Add : Sum
  Add1 : Sum  Inputs=-+
  Add10 : Sum  Inputs=-+
  Add2 : Sum  Inputs=+-
  Add4 : Sum  Inputs=-+
  Add5 : Sum  Inputs=+++
  Add6 : Sum  Inputs=+-
  Add8 : Sum  Inputs=+++
  Add9 : Sum  Inputs=+-
  Constant : Constant  Value=1.0
  Constant1 : Constant  Value=1.0
  Constant2 : Constant  Value=7/9
  Constant3 : Constant  Value=1.2
  Constant4 : Constant  Value=1.5
  Constant5 : Constant  Value=1.5
  Constant6 : Constant  Value=1.2
  Constant7 : Constant  Value=2.0
  Constant8 : Constant  Value=2.0
  Constant9 : Constant  Value=3
  Divide : Product  Inputs=*/
  Gain : Gain  Gain=-1
  Math Function1 : Math  Operator=pow  SignedPower=on  SaturateOnIntegerOverflow=on
  Product{1,3..9} (8 alike) : Product
  utx : Outport
  wires:
  Product9/1 -> Add8/2
  Product8/1 -> Add8/1
  Add9/1 -> Product9/1
  Constant6/1 -> Product9/2
  Add10/1 -> Product8/2
  Constant5/1 -> Product8/1
  Add8/1 -> Product1/2
  Product4/1 -> Add5/2
  Product5/1 -> Add5/3
  Constant4/1 -> Product4/1
  Add4/1 -> Product4/2
  xx6/1 -> Add1/2, Add2/1, Add4/2
  Constant3/1 -> Product5/2
  Product6/1 -> Add/1
  Constant/1 -> Product6/1
  Constant1/1 -> Product1/1
  Product1/1 -> Add/2
  Add2/1 -> Product5/1
  Add5/1 -> Product6/2
  xx2/1 -> Add4/1
  xx1/1 -> Add2/2
  vx1/1 -> Add9/2
  vx2/1 -> Add10/1
  vx6/1 -> Add6/1, Add9/1, Add10/2
  xx0/1 -> Add1/1
  Constant7/1 -> Product3/1
  Add1/1 -> Product3/2
  Product3/1 -> Add5/1
  vx0/1 -> Add6/2
  Constant8/1 -> Product7/2
  Add6/1 -> Product7/1
  Product7/1 -> Add8/3
  Math Function1/1 -> Gain/1
  Constant9/1 -> Divide/2
  Divide/1 -> Math Function1/1
  Add/1 -> Divide/1
  Constant2/1 -> Math Function1/2
  Gain/1 -> utx/1

== system chap04_CA2/Subsystem/Subsystem4/Subsystem7 ==
  vy6 : Inport
  vy0 : Inport  Port=2
  uty : Inport  Port=3
  gain : Inport  Port=4
  Add1 : Sum  Inputs=--+
  Constant : Constant  Value=0.08
  Constant2 : Constant  Value=15
  Product : Product
  Product1 : Product
  Product2 : Product
  Subsystem : Subsystem
  Subtract : Sum  Inputs=+--
  Tanh : Trigonometry  Operator=tanh
  ux : Outport
  wires:
  Subtract/1 -> Product2/1, Product1/2
  Constant/1 -> Product1/1
  Product1/1 -> Add1/1
  Constant2/1 -> Product2/2
  [A] -> Add1/3
  gain/1 -> Product/2
  Tanh/1 -> Product/1
  Product2/1 -> Tanh/1
  vy6/1 -> Subtract/1
  Product/1 -> Add1/2
  Subsystem/1(Out1) -> Subtract/3
  uty/1 -> Subsystem/1(zt3), [A]
  Add1/1 -> ux/1
  vy0/1 -> Subtract/2

== system chap04_CA2/Subsystem/Subsystem4/Subsystem8 ==
  vz6 : Inport
  vz0 : Inport  Port=2
  utz : Inport  Port=3
  gain : Inport  Port=4
  Add1 : Sum  Inputs=--+
  Constant : Constant  Value=0.08
  Constant2 : Constant  Value=15
  Product : Product
  Product1 : Product
  Product2 : Product
  Subsystem : Subsystem
  Subtract : Sum  Inputs=+--
  Tanh : Trigonometry  Operator=tanh
  ux : Outport
  wires:
  Add1/1 -> ux/1
  utz/1 -> [A], Subsystem/1(zt3)
  Subsystem/1(Out1) -> Subtract/3
  Product/1 -> Add1/2
  vz6/1 -> Subtract/1
  Product2/1 -> Tanh/1
  Tanh/1 -> Product/1
  gain/1 -> Product/2
  [A] -> Add1/3
  Constant2/1 -> Product2/2
  Product1/1 -> Add1/1
  Constant/1 -> Product1/1
  Subtract/1 -> Product1/2, Product2/1
  vz0/1 -> Subtract/2

== system chap04_CA2/Subsystem/Subsystem5/Subsystem1 ==
  xy3 : Inport
  xy1 : Inport  Port=2
  xy4 : Inport  Port=3
  xy5 : Inport  Port=4
  vy3 : Inport  Port=5
  vy1 : Inport  Port=6
  vy4 : Inport  Port=7
  vy5 : Inport  Port=8
  Add : Sum
  Add{1,4,6,8} (4 alike) : Sum  Inputs=-+
  Add2 : Sum  Inputs=+-
  Add5 : Sum  Inputs=+++
  Add7 : Sum  Inputs=+-
  Add9 : Sum  Inputs=+++
  Constant{,1,3,6} (4 alike) : Constant  Value=1.0
  Constant2 : Constant  Value=7/9
  Constant4 : Constant  Value=0.5
  Constant5 : Constant  Value=1.5
  Constant7 : Constant  Value=0.5
  Constant8 : Constant  Value=1.5
  Constant9 : Constant  Value=3
  Divide : Product  Inputs=*/
  Gain : Gain  Gain=-1
  Math Function1 : Math  Operator=pow  SignedPower=on  SaturateOnIntegerOverflow=on
  Product{1,3..9} (8 alike) : Product
  p3y : Outport
  wires:
  Add9/1 -> Product1/2
  Product4/1 -> Add5/2
  Product5/1 -> Add5/3
  Constant3/1 -> Product4/1
  Add4/1 -> Product4/2
  xy3/1 -> Add1/2, Add4/2, Add2/1
  Constant4/1 -> Product5/2
  Product6/1 -> Add/1
  Constant/1 -> Product6/1
  Constant1/1 -> Product1/1
  Product1/1 -> Add/2
  Add2/1 -> Product5/1
  Add5/1 -> Product6/2
  xy4/1 -> Add4/1
  xy1/1 -> Add2/2
  xy5/1 -> Add1/1
  Constant5/1 -> Product3/1
  Add1/1 -> Product3/2
  Product3/1 -> Add5/1
  Product7/1 -> Add9/1
  Add6/1 -> Product7/2
  Constant8/1 -> Product7/1
  vy5/1 -> Add6/1
  vy1/1 -> Add7/2
  vy4/1 -> Add8/1
  Add7/1 -> Product9/1
  Constant7/1 -> Product9/2
  vy3/1 -> Add7/1, Add8/2, Add6/2
  Add8/1 -> Product8/2
  Constant6/1 -> Product8/1
  Product9/1 -> Add9/3
  Product8/1 -> Add9/2
  Math Function1/1 -> Gain/1
  Constant9/1 -> Divide/2
  Divide/1 -> Math Function1/1
  Add/1 -> Divide/1
  Constant2/1 -> Math Function1/2
  Gain/1 -> p3y/1

== system chap04_CA2/Subsystem/Subsystem5/Subsystem10 ==
  utx : Inport
  uty : Inport  Port=2
  utz : Inport  Port=3
  Add : Sum
  Constant3 : Constant
  Constant4 : Constant  Value=0
  Data Store Memory : DataStoreMemory  DataStoreName=utkz3  ReadBeforeWriteMsg=warning  WriteAfterWriteMsg=warning  WriteAfterReadMsg=warning  ShowAdditionalParam=off
  Data Store Memory1 : DataStoreMemory  DataStoreName=utky3  ReadBeforeWriteMsg=warning  WriteAfterWriteMsg=warning  WriteAfterReadMsg=warning  ShowAdditionalParam=off
  Data Store Memory2 : DataStoreMemory  DataStoreName=utkx3  ReadBeforeWriteMsg=warning  WriteAfterWriteMsg=warning  WriteAfterReadMsg=warning  ShowAdditionalParam=off
  Data Store Memory3 : DataStoreMemory  DataStoreName=uc3  ReadBeforeWriteMsg=warning  WriteAfterWriteMsg=warning  WriteAfterReadMsg=warning  ShowAdditionalParam=off
  Data Store Read : DataStoreRead  DataStoreName=uc3  IndexOptions=Index vector (dialog)  Indices=1  OutputSizes=1
  Data Store Read4 : DataStoreRead  DataStoreName=utky3  IndexOptions=Index vector (dialog)  Indices=1  OutputSizes=1
  Data Store Read5 : DataStoreRead  DataStoreName=utkz3  IndexOptions=Index vector (dialog)  Indices=1  OutputSizes=1
  Data Store Read6 : DataStoreRead  DataStoreName=utkx3  IndexOptions=Index vector (dialog)  Indices=1  OutputSizes=1
  Data Store Write : DataStoreWrite  DataStoreName=uc3  IndexOptions=Index vector (dialog)  Indices=1  OutputSizes=1
  Data Store Write1 : DataStoreWrite  DataStoreName=utkx3  IndexOptions=Index vector (dialog)  Indices=1  OutputSizes=1
  Data Store Write2 : DataStoreWrite  DataStoreName=utky3  IndexOptions=Index vector (dialog)  Indices=1  OutputSizes=1
  Data Store Write3 : DataStoreWrite  DataStoreName=utkz3  IndexOptions=Index vector (dialog)  Indices=1  OutputSizes=1
  Demux : Demux  Outputs=3
  Display : Display
  MATLAB Function : MATLAB Function  TreatAsAtomicUnit=on
  Mux1 : Mux  Inputs=3
  Mux2 : Mux  Inputs=3
  Switch : Switch  Threshold=0.025
  Switch2 : Switch  Threshold=0.025
  ux : Outport
  uy : Outport  Port=2
  uz : Outport  Port=3
  wires:
  Mux2/1 -> [utk], MATLAB Function/2(utk)
  Mux1/1 -> [ut], MATLAB Function/1(u)
  Switch/1 -> Demux/1
  Data Store Read6/1 -> Mux2/1
  Data Store Read5/1 -> Mux2/3
  Data Store Read4/1 -> Mux2/2
  Demux/3 -> Data Store Write3/1, uz/1
  Demux/1 -> Data Store Write1/1, ux/1
  Add/1 -> Data Store Write/1, Display/1
  Data Store Read/1 -> Add/2
  Switch2/1 -> Add/1  "e1"
  Constant3/1 -> Switch2/1
  Constant4/1 -> Switch2/3
  MATLAB Function/1(nrom) -> Switch2/2, Switch/2
  utx/1 -> Mux1/1
  uty/1 -> Mux1/2
  utz/1 -> Mux1/3
  Demux/2 -> Data Store Write2/1, uy/1
  [ut] -> Switch/1
  [utk] -> Switch/3

== system chap04_CA2/Subsystem/Subsystem5/Subsystem2 ==
  xz3 : Inport
  xz1 : Inport  Port=2
  xz4 : Inport  Port=3
  xz5 : Inport  Port=4
  vz3 : Inport  Port=5
  vz1 : Inport  Port=6
  vz4 : Inport  Port=7
  vz5 : Inport  Port=8
  Add : Sum
  Add{1,4,6,8} (4 alike) : Sum  Inputs=-+
  Add2 : Sum  Inputs=+-
  Add5 : Sum  Inputs=+++
  Add7 : Sum  Inputs=+-
  Add9 : Sum  Inputs=+++
  Constant{,1,3,6} (4 alike) : Constant  Value=1.0
  Constant2 : Constant  Value=7/9
  Constant4 : Constant  Value=0.5
  Constant5 : Constant  Value=1.5
  Constant7 : Constant  Value=0.5
  Constant8 : Constant  Value=1.5
  Constant9 : Constant  Value=3
  Divide : Product  Inputs=*/
  Gain : Gain  Gain=-1
  Math Function1 : Math  Operator=pow  SignedPower=on  SaturateOnIntegerOverflow=on
  Product{1,3..9} (8 alike) : Product
  p3z : Outport
  wires:
  Product8/1 -> Add9/2
  Product9/1 -> Add9/3
  Constant6/1 -> Product8/1
  Add8/1 -> Product8/2
  vz3/1 -> Add6/2, Add8/2, Add7/1
  Constant7/1 -> Product9/2
  Add7/1 -> Product9/1
  vz4/1 -> Add8/1
  vz1/1 -> Add7/2
  vz5/1 -> Add6/1
  Constant8/1 -> Product7/1
  Add6/1 -> Product7/2
  Product7/1 -> Add9/1
  Product3/1 -> Add5/1
  Add1/1 -> Product3/2
  Constant5/1 -> Product3/1
  xz5/1 -> Add1/1
  xz1/1 -> Add2/2
  xz4/1 -> Add4/1
  Add5/1 -> Product6/2
  Add2/1 -> Product5/1
  Product1/1 -> Add/2
  Constant1/1 -> Product1/1
  Constant/1 -> Product6/1
  Product6/1 -> Add/1
  Constant4/1 -> Product5/2
  xz3/1 -> Add2/1, Add4/2, Add1/2
  Add4/1 -> Product4/2
  Constant3/1 -> Product4/1
  Product5/1 -> Add5/3
  Product4/1 -> Add5/2
  Add9/1 -> Product1/2
  Math Function1/1 -> Gain/1
  Constant9/1 -> Divide/2
  Divide/1 -> Math Function1/1
  Add/1 -> Divide/1
  Constant2/1 -> Math Function1/2
  Gain/1 -> p3z/1

== system chap04_CA2/Subsystem/Subsystem5/Subsystem4 ==
  vx3 : Inport
  utx : Inport  Port=2
  gain : Inport  Port=3
  Add1 : Sum  Inputs=--+
  Constant : Constant  Value=0.08
  Constant2 : Constant  Value=15
  Product : Product
  Product1 : Product
  Product2 : Product
  Subsystem : Subsystem
  Subtract : Sum  Inputs=+-
  Tanh : Trigonometry  Operator=tanh
  ux : Outport
  wires:
  Add1/1 -> ux/1
  utx/1 -> [A], Subsystem/1(zt3)
  Subsystem/1(Out1) -> Subtract/2
  Product/1 -> Add1/2
  vx3/1 -> Subtract/1
  Product2/1 -> Tanh/1
  Tanh/1 -> Product/1
  gain/1 -> Product/2
  [A] -> Add1/3
  Constant2/1 -> Product2/2
  Product1/1 -> Add1/1
  Constant/1 -> Product1/1
  Subtract/1 -> Product1/2, Product2/1
